simulink model "bdc_motor_sim"  (R2025b)
settings: Solver=VariableStepAuto  StartTime=0.0  StopTime=10  RelTol=1e-3
values from neighbouring files (symbols this model uses):
  A = [-Ra/La, -K/La; K/Je, -Be/Je]    [bdc_motor_src.m]
  B = [1/La; 0]    [bdc_motor_src.m]
  Be = 0.1    [bdc_motor_src.m]
  C = [0, 1]    [bdc_motor_src.m]
  D = 0    [bdc_motor_src.m]
  den = [(Je*La), (Je*Ra + Be*La), (Be*Ra + K^2)]    [bdc_motor_src.m]
  Je = 0.01    [bdc_motor_src.m]
  K = 0.01    [bdc_motor_src.m]
  La = 0.5    [bdc_motor_src.m]
  num = K    (= 0.01)    [bdc_motor_src.m]
  Ra = 0.5    [bdc_motor_src.m]
settings Model: LastModifiedBy=maxvega

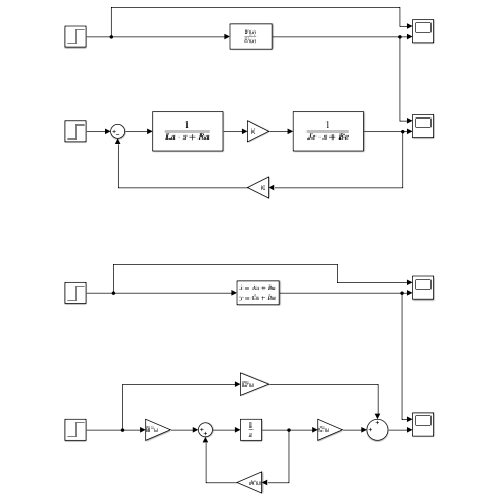
[thumbnail: Simulink's stored preview of the top-level diagram]
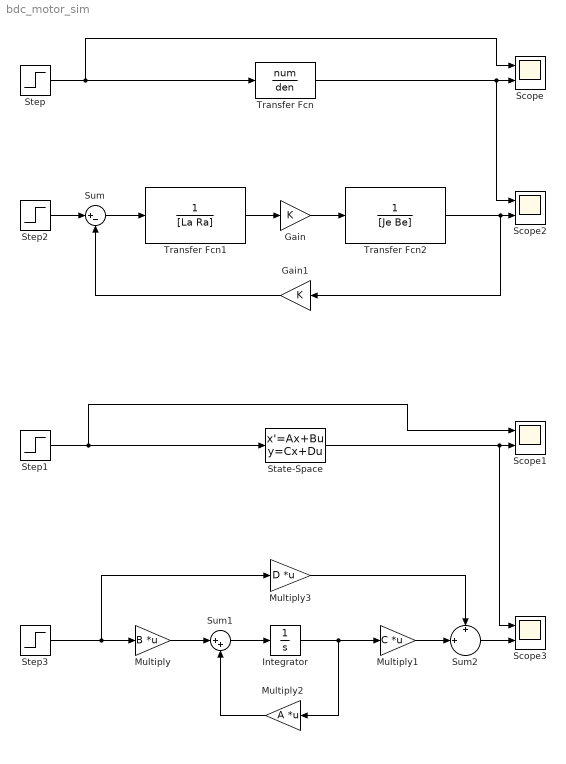
== system bdc_motor_sim ==
  Gain : Gain  Gain=K
  Gain1 : Gain  Gain=K
  Integrator : Integrator
  Multiply : Gain  Gain=B  Multiplication=Matrix(K*u)
  Multiply1 : Gain  Gain=C  Multiplication=Matrix(K*u)
  Multiply2 : Gain  Gain=A  Multiplication=Matrix(K*u)
  Multiply3 : Gain  Gain=D  Multiplication=Matrix(K*u)
  Scope{,1..3} (4 alike) : Scope  NumInputPorts=2
      Scope settings: ActiveDisplayYMinimum=-0.125  ActiveDisplayYMaximum=1.125
      Scope1 settings: ActiveDisplayYMinimum=-0.125  ActiveDisplayYMaximum=1.125
      Scope2 settings: ActiveDisplayYMinimum=-0.02495  ActiveDisplayYMaximum=0.22452  DataLoggingVariableName=ScopeData2
      Scope3 settings: ActiveDisplayYMinimum=-0.02495  ActiveDisplayYMaximum=0.22452  DataLoggingVariableName=ScopeData3
  State-Space : StateSpace  A=A  B=B  C=C  D=D  InitialCondition=0
  Step{,1..3} (4 alike) : Step  SampleTime=0
  Sum : Sum  Inputs=|+-
  Sum1 : Sum  Inputs=|++
  Sum2 : Sum  Inputs=+|+||
  Transfer Fcn : TransferFcn  Numerator=num  Denominator=den
  Transfer Fcn1 : TransferFcn  Denominator=[La Ra]
  Transfer Fcn2 : TransferFcn  Denominator=[Je Be]
  wires:
  Transfer Fcn/1 -> Scope/2, Scope2/1
  Step/1 -> Transfer Fcn/1, Scope/1
  Step1/1 -> Scope1/1, State-Space/1
  Transfer Fcn2/1 -> Scope2/2, Gain1/1
  Step2/1 -> Sum/1
  Gain1/1 -> Sum/2
  Sum/1 -> Transfer Fcn1/1
  Transfer Fcn1/1 -> Gain/1
  Gain/1 -> Transfer Fcn2/1
  State-Space/1 -> Scope1/2, Scope3/1
  Multiply/1 -> Sum1/1
  Sum1/1 -> Integrator/1
  Multiply2/1 -> Sum1/2
  Integrator/1 -> Multiply1/1, Multiply2/1
  Sum2/1 -> Scope3/2
  Step3/1 -> Multiply3/1, Multiply/1
  Multiply1/1 -> Sum2/2
  Multiply3/1 -> Sum2/1
